simulink model "gm_main"  (R2022b)
settings: Solver=FixedStepDiscrete  StartTime=0.0  StopTime=4050e-6  RelTol=1e-3
libraries: simulink x2, hdlsllib x1
settings Model: Creator=mella  LastModifiedBy=mella
settings SolverCC: AlgebraicLoopSolver=TrustRegion
settings DataIOCC: LimitDataPoints=on  SaveOutput=off  SaveTime=off
settings OptimizationCC: BlockReduction=off  ConditionallyExecuteInputs=off  DefaultParameterBehavior=Inlined  LifeSpan=inf
settings DebuggingCC: AlgebraicLoopMsg=error  InheritedTsInSrcMsg=none  SingleTaskRateTransMsg=error  UnconnectedInputMsg=warning  UnconnectedOutputMsg=warning  UnconnectedLineMsg=warning  AllowSymbolicDim=off  StrictBusMsg=ErrorOnBusTreatedAsVector  SFUnexpectedBacktrackingDiag=warning  SFNoUnconditionalDefaultTransitionDiag=warning  SFExecutionAtInitializationDiag=none  SFMachineParentedDataDiag=warning  ArithmeticOperatorsInVariantConditions=warning
settings HardwareCC: ProdBitPerPointer=32  ProdBitPerSizeT=32  ProdBitPerPtrDiffT=32  ProdLargestAtomicFloat=None  ProdIntDivRoundTo=Undefined  ProdEndianess=Unspecified  ProdWordSize=32  ProdHWDeviceType=ASIC/FPGA->ASIC/FPGA  ProdEqTarget=off
settings ModelReferenceCC: EnableRefExpFcnMdlSchedulingChecks=on
settings SFSimCC: SimUseLocalCustomCode=off  CustomCodeUndefinedFunction=UseInterfaceOnly
settings RTWCC: RTWUseLocalCustomCode=off
settings CodeAppCC: StateflowObjectComments=on
settings GRTTargetCC: TargetLangStandard=C89/C90 (ANSI)
settings ConfigComp: CovScope=ReferencedModels  CovMetricSettings=dw  CovSaveCumulativeToWorkspaceVar=on  CovSaveSingleToWorkspaceVar=on  CovExternalEMLEnable=off  CovSFcnEnable=off

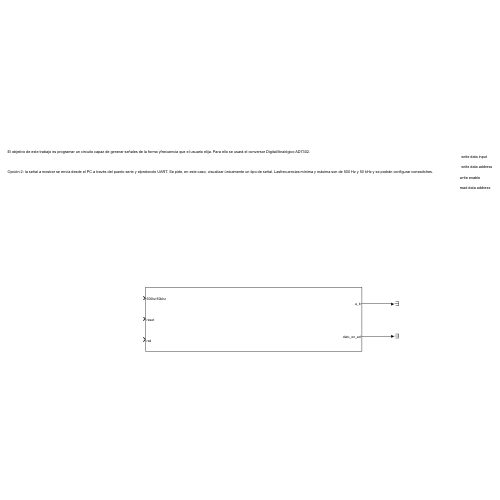
[thumbnail: Simulink's stored preview of the top-level diagram]
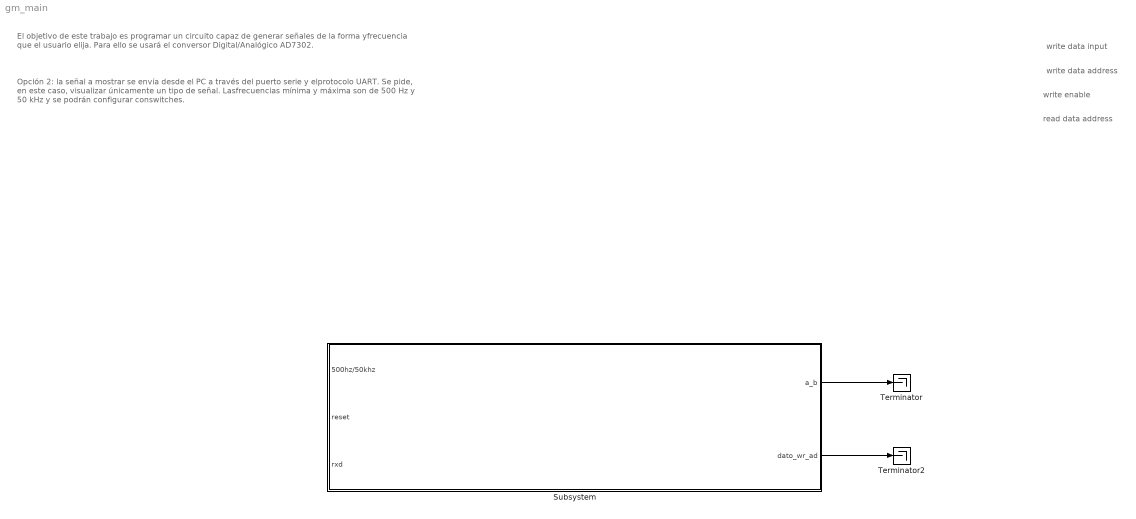
== system gm_main ==
  note: read data address
  note: write enable
  note: write data address
  note: write data input
  note: Opción 2: la señal a mostrar se envía desde el PC a través del puerto serie y elprotocolo UART. Se pide, en este caso, visualizar únicamente un tipo de señal. Lasfrecuencias mínima y máxima son de 500 Hz y 50 kHz y se podrán configurar conswitches.
  note: El objetivo de este trabajo es programar un circuito capaz de generar señales de la forma yfrecuencia que el usuario elija. Para ello se usará el conversor Digital/Analógico AD7302.
  Subsystem : Subsystem
  Terminator : Terminator
  Terminator2 : Terminator
  wires:
  Subsystem/2(dato_wr_ad) -> Terminator2/1
  Subsystem/1(a_b) -> Terminator/1

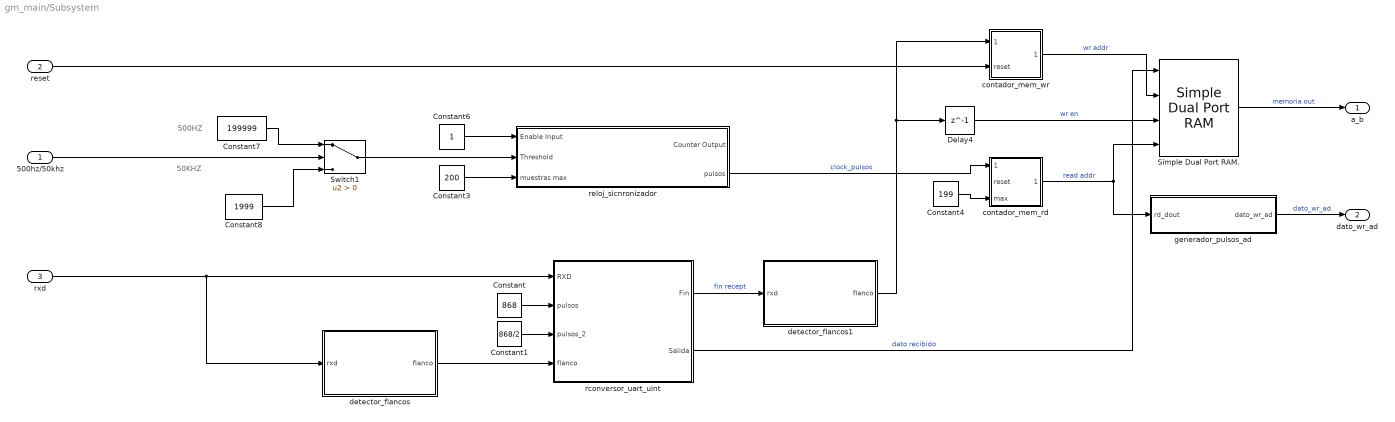
== system gm_main/Subsystem ==
  note: 500HZ
  note: 50KHZ
  500hz/50khz : Inport  OutDataTypeStr=boolean
  reset : Inport  Port=2
  rxd : Inport  Port=3
  Constant : Constant  Value=868  OutDataTypeStr=fixdt(0,16,0)
  Constant1 : Constant  Value=868/2  OutDataTypeStr=fixdt(0,16,0)
  Constant3 : Constant  Value=200  OutDataTypeStr=uint32
  Constant4 : Constant  Value=199  OutDataTypeStr=uint8
  Constant6 : Constant  OutDataTypeStr=boolean
  Constant7 : Constant  Value=199999  OutDataTypeStr=uint32  SampleTime=10e-9
  Constant8 : Constant  Value=1999  OutDataTypeStr=uint32  SampleTime=10e-9
  Delay4 : Delay  DelayLength=1
  Simple Dual Port RAM. : hdlsllib/HDL RAMs/Simple Dual Port RAM  ram_size=8
  Switch1 : Switch  Criteria=u2 > Threshold  SaturateOnIntegerOverflow=off  InputSameDT=off
  contador_mem_rd : Stateflow chart  TreatAsAtomicUnit=on
  contador_mem_wr : Stateflow chart  TreatAsAtomicUnit=on
  detector_flancos : Subsystem
  detector_flancos1 : Subsystem
  generador_pulsos_ad : Subsystem  TreatAsAtomicUnit=on
  rconversor_uart_uint : Stateflow chart  TreatAsAtomicUnit=on
      settings: PortSchema="{\"entries\":[{\"content\":{\"sides\":[{\"content\":{\"connectorIds\":[\"In3\",\"In1\",\"In2\",\"In4\"]},\"type\":\"ConnectorPlacement.EquallySpacedRectSide\",\"uuid\":\"def6cf29-dd98-4e60-b4e2-f9a28f4e0216\"},{\"content\":{\"connectorIds\":[\"Out1\",\"Out2\"],\"side\":\"RIGHT\"},\"type\":\"ConnectorPlacement.EquallySpacedRectSide\",\"uuid\":\"357314fe-5b9a-42b5-a119-47ec938df135\"},{\"content\":{\"connectorIds\":[],\"side\":\"TOP\"},\"type\":\"ConnectorPlacement.EquallySpacedRectSide\",\"uuid\":\"54a71f5f-36eb-4905-951f-0137ad009dd2\"},{\"content\":{\"connectorIds\":[],\"side\":\"BOTTOM\"},\"type\":\"ConnectorPlacement.EquallySpacedRectSide\",\"uuid\":\"d2f3902b-eb7b-4794-adfd-f8c054305e62\"}]},\"type\":\"ConnectorPlacement.EquallySpacedConnector\",\"uuid\":\"9e015aad-694e-4ed2-84a8-f955325fe360\"}],\"packageUris\":[\"http://schema.mathworks.com/mf0/Connector/R2020b\"],\"version\":\"1.0\"}"
  reloj_sicnronizador : Subsystem
  a_b : Outport
  dato_wr_ad : Outport  Port=2
  wires:
  detector_flancos/1(flanco) -> rconversor_uart_uint/4(flanco)
  generador_pulsos_ad/1(dato_wr_ad) -> dato_wr_ad/1  "dato_wr_ad"
  Simple Dual Port RAM./1 -> a_b/1  "memoria out"
  Constant4/1 -> contador_mem_rd/3(max)
  contador_mem_rd/1(salida) -> generador_pulsos_ad/1(rd_dout), Simple Dual Port RAM./4  "read addr"
  Constant3/1 -> reloj_sicnronizador/3(muestras max)
  reloj_sicnronizador/2(pulsos) -> contador_mem_rd/1(sumar)  "clock_pulsos"
  Constant8/1 -> Switch1/3
  rxd/1 -> rconversor_uart_uint/3(RXD), detector_flancos/1(rxd)
  detector_flancos1/1(flanco) -> contador_mem_wr/1(sumar), Delay4/1
  Constant1/1 -> rconversor_uart_uint/2(pulsos_2)
  rconversor_uart_uint/1(Fin) -> detector_flancos1/1(rxd)  "fin recept"
  500hz/50khz/1 -> Switch1/2
  Switch1/1 -> reloj_sicnronizador/2(Threshold)
  Constant7/1 -> Switch1/1
  reset/1 -> contador_mem_wr/2(reset)
  Delay4/1 -> Simple Dual Port RAM./3  "wr en"
  contador_mem_wr/1(salida) -> Simple Dual Port RAM./2  "wr addr"
  Constant/1 -> rconversor_uart_uint/1(pulsos)
  Constant6/1 -> reloj_sicnronizador/1(Enable Input)
  rconversor_uart_uint/2(Salida) -> Simple Dual Port RAM./1  "dato recibido"

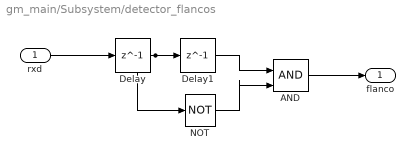
== system gm_main/Subsystem/detector_flancos ==
  rxd : Inport
  AND : Logic  IconShape=distinctive  AllPortsSameDT=off  OutDataTypeStr=boolean
  Delay : Delay  DelayLength=1
  Delay1 : Delay  DelayLength=1
  NOT : Logic  Operator=NOT  IconShape=distinctive  AllPortsSameDT=off  OutDataTypeStr=boolean
  flanco : Outport
  wires:
  rxd/1 -> Delay/1
  AND/1 -> flanco/1
  Delay/1 -> Delay1/1, NOT/1
  Delay1/1 -> AND/1
  NOT/1 -> AND/2

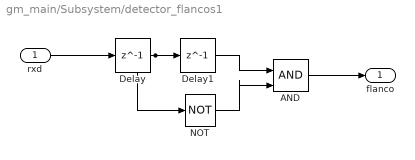
== system gm_main/Subsystem/detector_flancos1 ==
  rxd : Inport
  AND : Logic  IconShape=distinctive  AllPortsSameDT=off  OutDataTypeStr=boolean
  Delay : Delay  DelayLength=1
  Delay1 : Delay  DelayLength=1
  NOT : Logic  Operator=NOT  IconShape=distinctive  AllPortsSameDT=off  OutDataTypeStr=boolean
  flanco : Outport
  wires:
  rxd/1 -> Delay/1
  AND/1 -> flanco/1
  Delay/1 -> Delay1/1, NOT/1
  Delay1/1 -> AND/1
  NOT/1 -> AND/2

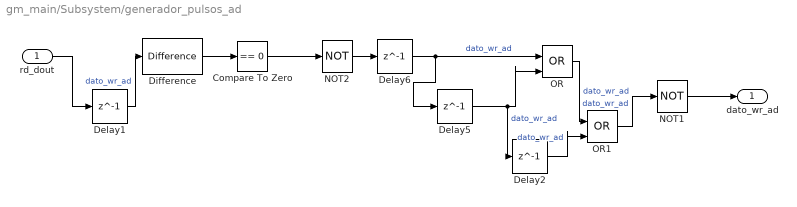
== system gm_main/Subsystem/generador_pulsos_ad ==
  rd_dout : Inport
  Compare To Zero : simulink/Logic and Bit Operations/Compare To Zero  relop===  OutDataTypeStr=boolean
  Delay{1..2,5..6} (4 alike) : Delay  DelayLength=1
  Difference : simulink/Discrete/Difference  ICPrevInput=0.0  OutMin=[]  OutMax=[]  OutDataType=fixdt(1, 16)  OutScaling=2^-10  DoSatur=off
  NOT1 : Logic  Operator=NOT  IconShape=distinctive  AllPortsSameDT=off  OutDataTypeStr=boolean
  NOT2 : Logic  Operator=NOT  IconShape=distinctive  AllPortsSameDT=off  OutDataTypeStr=boolean
  OR : Logic  Operator=OR  IconShape=distinctive  AllPortsSameDT=off  OutDataTypeStr=boolean
  OR1 : Logic  Operator=OR  IconShape=distinctive  AllPortsSameDT=off  OutDataTypeStr=boolean
  dato_wr_ad : Outport
  wires:
  Delay1/1 -> Difference/1  "dato_wr_ad"
  Delay2/1 -> OR1/2  "dato_wr_ad"
  OR1/1 -> NOT1/1  "dato_wr_ad"
  NOT1/1 -> dato_wr_ad/1
  rd_dout/1 -> Delay1/1
  OR/1 -> OR1/1  "dato_wr_ad"
  Difference/1 -> Compare To Zero/1
  Compare To Zero/1 -> NOT2/1
  NOT2/1 -> Delay6/1
  Delay5/1 -> OR/2, Delay2/1  "dato_wr_ad"
  Delay6/1 -> Delay5/1, OR/1  "dato_wr_ad"

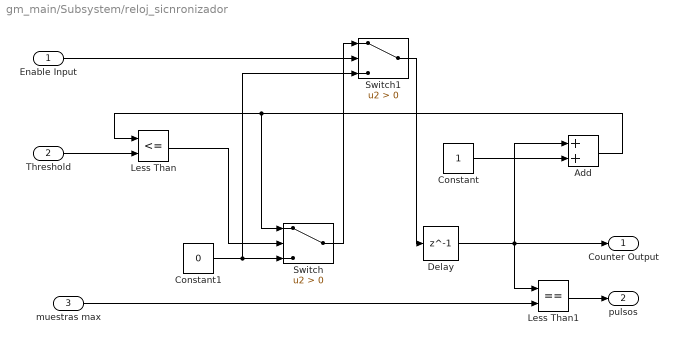
== system gm_main/Subsystem/reloj_sicnronizador ==
  Enable Input : Inport  OutDataTypeStr=boolean
  Threshold : Inport  Port=2  OutDataTypeStr=uint32
  muestras max : Inport  Port=3
  Add : Sum  OutDataTypeStr=uint16
  Constant : Constant  OutDataTypeStr=uint32  SampleTime=-1
  Constant1 : Constant  Value=0  OutDataTypeStr=uint32  SampleTime=-1
  Delay : Delay  DelayLength=1
  Less Than : RelationalOperator  Operator=<=  OutDataTypeStr=boolean  RndMeth=Simplest  InputSameDT=off
  Less Than1 : RelationalOperator  Operator===  OutDataTypeStr=boolean  RndMeth=Simplest  InputSameDT=off
  Switch : Switch  Criteria=u2 > Threshold  SaturateOnIntegerOverflow=off  InputSameDT=off
  Switch1 : Switch  Criteria=u2 > Threshold  SaturateOnIntegerOverflow=off  InputSameDT=off
  Counter Output : Outport  OutDataTypeStr=uint32  VectorParamsAs1DForOutWhenUnconnected=off
  pulsos : Outport  Port=2
  wires:
  Enable Input/1 -> Switch1/2
  Constant1/1 -> Switch/3, Switch1/3
  Add/1 -> Switch/1, Less Than/1
  Delay/1 -> Add/1, Counter Output/1, Less Than1/1
  Less Than/1 -> Switch/2
  Constant/1 -> Add/2
  Switch1/1 -> Delay/1
  muestras max/1 -> Less Than1/2
  Threshold/1 -> Less Than/2
  Switch/1 -> Switch1/1
  Less Than1/1 -> pulsos/1

== stateflow chart gm_main/Subsystem/contador_mem_rd ==
  settings: stateMachineType=MOORE_MACHINE  initializeOutput=1
  state inicio
    cont=0;
  state Reset
    cont=0;
    salida=cont;
  state Espera
    salida=cont;
  state incrementa
    salida=cont;
  (default) -> inicio
  inicio -> Espera
  Espera -> Espera [order 3]
  Reset -> Espera : [after(1,tick)]
  incrementa -> Espera [order 3] : [after(1,tick)]{cont=cont+1;}
  Espera -> incrementa [order 2] : [sumar==true]
  Espera -> Reset [order 1] : [reset==1]
  incrementa -> Reset [order 2] : [cont==max]
  incrementa -> Reset [order 1] : [reset==1]
  data: sumar input boolean; salida output uint8; cont local uint8; reset input boolean; max input

== stateflow chart gm_main/Subsystem/rconversor_uart_uint ==
  settings: stateMachineType=MOORE_MACHINE  executeAtInitialization=1  initializeOutput=1
  state e_inicio
    Fin = false;
    Intermedio = 0;
    salidaAux = 0;
    Salida = 0
    i = 0
  state E_espera
    Intermedio = 0;
    i = 0
    Fin = false;
    Salida = salidaAux;
    i = 0;
  state e_rota
    Fin = false;
    Salida = salidaAux;
    Intermedio = bitconcat(RXD,bitsliceget(Intermedio,8,2))
  state e_fin
    Fin = true;
    salidaAux = Intermedio;
    Salida = salidaAux;
  state E_espera2
    Fin = false;
    Salida = salidaAux;
  state e_reposo
    Fin = false;
    Salida = salidaAux;
  (default) -> e_inicio
  e_inicio -> E_espera : [flanco==true]
  e_rota -> e_fin [order 2]
  E_espera -> E_espera2 : [after(pulsos_2,tick)]
  E_espera2 -> e_rota : [after(pulsos,tick)]
  e_fin -> e_reposo
  e_rota -> E_espera2 [order 1] : [i<7]{i=i+1}
  e_reposo -> E_espera [order 1] : [flanco==true]
  e_reposo -> e_reposo [order 2]
  data: pulsos input fixdt(0,16,0); pulsos_2 input; RXD input fixdt(0,1,0); flanco input; Fin output boolean; Salida output fixdt(0,8,0); Intermedio local fixdt(0,8,0); i local uint16; salidaAux local fixdt(0,8,0)

== stateflow chart gm_main/Subsystem/contador_mem_wr ==
  settings: stateMachineType=MOORE_MACHINE  initializeOutput=1
  state inicio
    cont=0;
  state Reset
    cont=0;
    salida=cont;
  state Espera
    salida=cont;
  state incrementa
    salida=cont;
  (default) -> inicio
  inicio -> Espera
  Espera -> Espera [order 3]
  Reset -> Espera : [after(1,tick)]
  incrementa -> Espera [order 3] : [after(1,tick)]{cont=cont+1;}
  Espera -> incrementa [order 2] : [sumar==true]
  Espera -> Reset [order 1] : [reset==1]
  incrementa -> Reset [order 2] : [cont==199]
  incrementa -> Reset [order 1] : [reset==1]
  data: sumar input boolean; salida output uint8; cont local uint8; reset input boolean
